simulink model "VSC_GFo_Variable_Frequency_LCL_r2015a"  (R2015a)
settings: Solver=ode1  SolverMode=SingleTasking  StartTime=0.0  StopTime=8  FixedStep=Time_Step  MaxStep=1e-5  RelTol=1e-3
PreLoadFcn:
  | VSC_GFo_Init;
InitFcn:
  | VSC_GFo_Init;
values from neighbouring files (symbols this model uses):
  DX_DR = 5    [VSC_GFo_Init.m]
  fb = fn    (= 50)    [VSC_GFo_Init.m]    (also in VSC_GFo_Init_v1.m; VSC_GFo_Init_wi_LCL.m)
  fn = 50    [VSC_GFo_Init.m]    (also in VSC_GFo_Init_v1.m; VSC_GFo_Init_wi_LCL.m)
  GRD00_Lg = GRD00_Xg/wb    (= 0.0254647908947)    [VSC_GFo_Init.m]    (also in VSC_GFo_Init_v1.m; VSC_GFo_Init_wi_LCL.m)
  GRD00_Rg = GRD00_Rg_pu*GRD00_Zb    (= 0.8)    [VSC_GFo_Init.m]    (also in VSC_GFo_Init_v1.m; VSC_GFo_Init_wi_LCL.m)
  I_thresh_pu = 1    [VSC_GFo_Init.m]
  Kp_Rvi_pu = 0.676    [VSC_GFo_Init.m]
  Time_Step = 40e-6    (= 4e-05)    [VSC_GFo_Init.m]    (also in VSC_GFo_Init_v1.m; VSC_GFo_Init_wi_LCL.m)
  VSC01_Delta_P_Time_Step = 0.2    [VSC_GFo_Init.m]    (also in VSC_GFo_Init_v1.m; VSC_GFo_Init_wi_LCL.m)
  VSC01_Delta_P_Value = 0    [VSC_GFo_Init.m]    (also in VSC_GFo_Init_v1.m = 0.2; VSC_GFo_Init_wi_LCL.m = 0.2)
  VSC01_Udc_n = 640 * 1e3    (= 640000)    [VSC_GFo_Init.m]    (also in VSC_GFo_Init_v1.m; VSC_GFo_Init_wi_LCL.m)
  VSC01_Udcb = VSC01_Udc_n    (= 640000)    [VSC_GFo_Init.m]    (also in VSC_GFo_Init_v1.m; VSC_GFo_Init_wi_LCL.m)
undefined symbols (not defined in the file or in its folder): C_line, powergui, VSC01_id0
undefined symbols (not defined in the file): GRD00_H, GRD00_R, GRD00_TD, GRD00_TN, GRD00_Ub, VSC01_Cf, VSC01_Cf_pu, VSC01_Lf, VSC01_Lf_pu, VSC01_Lt_pu, VSC01_mp1, VSC01_mp2, VSC01_mp3, VSC01_Pn, VSC01_R, VSC01_Rf, VSC01_Rf_pu, VSC01_Rt_pu, VSC01_Rv, VSC01_Sn, VSC01_T1, VSC01_T2, VSC01_Tr_PLL, VSC01_Un1, VSC01_Un2, VSC01_W_LF, VSC01_wc1, VSC01_wc2, VSC01_wc3
libraries: powerlib x28, simulink x1, powerlib_meascontrol x1
(part 2 of 2)

== system VSC_GFo_Variable_Frequency_LCL_r2015a/VSC00/Control loops/Inner Cascaded control loops ==
  eg_dq0* : Inport
  eg_dq : Inport  Port=2
  ig_dq : Inport  Port=3
  is_dq : Inport  Port=4
  Amplitude : Subsystem
  Compare To Constant : simulink/Logic and Bit Operations/Compare To Constant  relop=<=  const=I_max  OutDataTypeStr=boolean
  Current PI control : Subsystem
      mask Display:
      | plot(0,0,100,100, [10,10,90,90,10,40,40,10,90,60,60,90],[90,10,10,90,90,60,40,10,10,40,60,90])
      | disp('PI')
  Memory : Memory
  Voltage PI control : Subsystem
      mask Display:
      | plot(0,0,100,100, [10,10,90,90,10,40,40,10,90,60,60,90],[90,10,10,90,90,60,40,10,10,40,60,90])
      | disp('PI')
  w_pu : Constant
  vm_dq : Outport
  wires:
  Amplitude/2(cond) -> Compare To Constant/1
  eg_dq0*/1 -> Voltage PI control/2(Eg_dq0*)
  Voltage PI control/1(Is_dq0*) -> Amplitude/1(is_unsat)
  Amplitude/1(is_sat) -> Current PI control/3(Is_dq0*)
  w_pu/1 -> Current PI control/4(w), Voltage PI control/4(w)
  Current PI control/1(Vm_dq0*) -> vm_dq/1
  is_dq/1 -> Current PI control/1(Is_dq0)
  eg_dq/1 -> Current PI control/2(Eg_dq0), Voltage PI control/1(Eg_dq0)
  ig_dq/1 -> Voltage PI control/3(Ig_dq0)
  Compare To Constant/1 -> Memory/1
  Memory/1 -> Voltage PI control/5(block integ)

== system VSC_GFo_Variable_Frequency_LCL_r2015a/VSC00/Control loops/PLL ==
  vg_abc_pu : Inport
  Demux : Demux  Outputs=2
  PI PLL controller : Subsystem
  Terminator : Terminator
  abc --> dq (normalized) : Subsystem
  delta_PLL : Outport
  w_PLL : Outport  Port=2
  wires:
  Demux/2 -> PI PLL controller/1(Vq)
  PI PLL controller/1(w_PLL) -> w_PLL/1
  Demux/1 -> Terminator/1
  PI PLL controller/2(delta_theta) -> abc --> dq (normalized)/2(Theta), delta_PLL/1
  vg_abc_pu/1 -> abc --> dq (normalized)/1(abc)
  abc --> dq (normalized)/1(dq) -> Demux/1

== system VSC_GFo_Variable_Frequency_LCL_r2015a/VSC00/Control loops/Power Control Loops ==
  P_mes : Inport
  P_set : Inport  Port=2
  delta_PLL : Inport  Port=3
  w_PLL : Inport  Port=4
  Merge : Merge  Inputs=3
  Merge1 : Merge  Inputs=3
  Power control loops : Subsystem
  Strategy 1 : Subsystem
  Strategy 2 : Subsystem
  Switch Case : SwitchCase  CaseConditions={1,2,3}  ShowDefaultCase=off
  w_set2 : Constant  Value=gainpopup
  w_set_pu : Constant
  f : Outport
  Theta : Outport  Port=2
  wires:
  w_set2/1 -> Switch Case/1
  P_mes/1 -> Power control loops/1(P_mes), Strategy 2/1(P_mes), Strategy 1/1(P_mes)
  P_set/1 -> Strategy 2/2(P_set), Power control loops/2(P_set), Strategy 1/2(P_set)
  delta_PLL/1 -> Strategy 1/3(delta_PLL)
  w_PLL/1 -> Strategy 2/3(w_PLL), Strategy 1/4(w_PLL)
  Switch Case/1 -> Strategy 1/Action
  Switch Case/2 -> Strategy 2/Action
  w_set_pu/1 -> Power control loops/3(w_set_pu)
  Switch Case/3 -> Power control loops/Action
  Strategy 1/1(frequency) -> Merge/1
  Strategy 2/1(frequency) -> Merge/2
  Power control loops/1(frequency) -> Merge/3
  Strategy 1/2(theta) -> Merge1/1
  Strategy 2/2(theta) -> Merge1/2
  Power control loops/2(theta) -> Merge1/3
  Merge/1 -> f/1
  Merge1/1 -> Theta/1

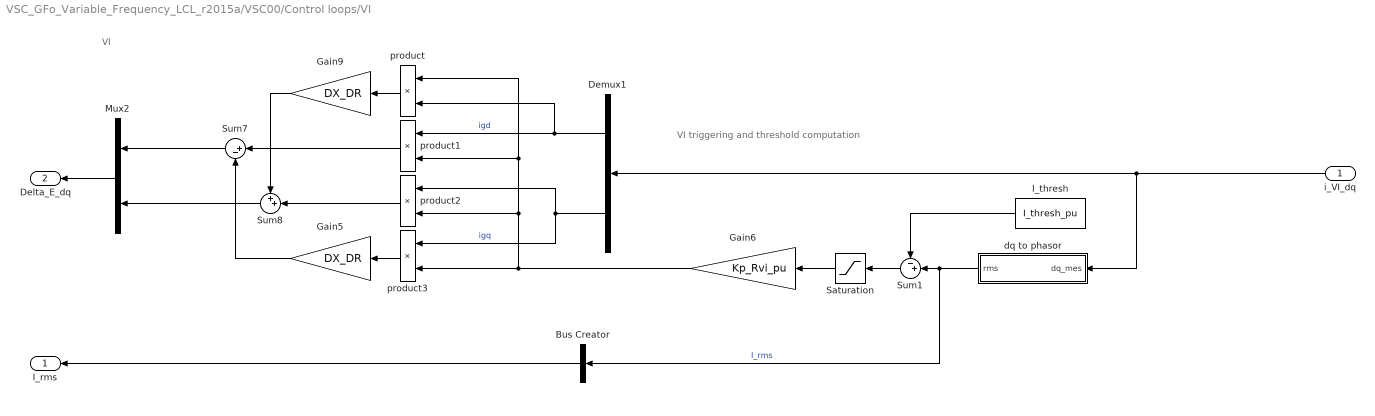
== system VSC_GFo_Variable_Frequency_LCL_r2015a/VSC00/Control loops/VI ==
  note: VI
  note: VI triggering and threshold computation
  i_VI_dq : Inport
  Bus Creator : BusCreator  Inputs=1
  Demux1 : Demux  Outputs=2
  Gain5 : Gain  Gain=DX_DR
  Gain6 : Gain  Gain=Kp_Rvi_pu
  Gain9 : Gain  Gain=DX_DR
  I_thresh : Constant  Value=I_thresh_pu
  Mux2 : Mux  Inputs=2
  Saturation : Saturate  UpperLimit=inf  LowerLimit=0
  Sum1 : Sum  Inputs=-+|
  Sum7 : Sum  Inputs=|+-
  Sum8 : Sum  Inputs=++|
  dq to phasor : Subsystem
  product{,1..3} (4 alike) : Product  SaturateOnIntegerOverflow=on  RndMeth=Zero  InputSameDT=on  OutDataTypeStr=Inherit: Same as first input
  I_rms : Outport
  Delta_E_dq : Outport  Port=2
  wires:
  i_VI_dq/1 -> Demux1/1, dq to phasor/1(dq_mes)
  Sum8/1 -> Mux2/2
  Sum7/1 -> Mux2/1
  product2/1 -> Sum8/2
  Gain9/1 -> Sum8/1
  Gain5/1 -> Sum7/2
  product1/1 -> Sum7/1
  Demux1/2 -> product3/1, product2/1  "igq"
  Demux1/1 -> product/2, product1/1  "igd"
  product/1 -> Gain9/1
  product3/1 -> Gain5/1
  Gain6/1 -> product2/2, product1/2, product/1, product3/2
  Mux2/1 -> Delta_E_dq/1
  I_thresh/1 -> Sum1/1
  Saturation/1 -> Gain6/1
  dq to phasor/1(rms) -> Bus Creator/1, Sum1/2  "I_rms"
  Sum1/1 -> Saturation/1
  Bus Creator/1 -> I_rms/1

== system VSC_GFo_Variable_Frequency_LCL_r2015a/VSC00/Control loops/abc --> dq (normalized) ==
  abc : Inport
  Theta : Inport  Port=2
  Demux3 : Demux  Outputs=3
  Mux2 : Mux  Inputs=2
  Normalization gain 1 pu rms in abc = 1 pu in dq : Gain  Gain=1/(sqrt(3))
  abc_2_alpha_beta : Subsystem
  alpha_beta_2_dq : Subsystem
  dq : Outport
  wires:
  Mux2/1 -> Normalization gain 1 pu rms in abc = 1 pu in dq/1
  abc_2_alpha_beta/1(alpha) -> alpha_beta_2_dq/2(a)
  Demux3/1 -> abc_2_alpha_beta/1(a)
  Demux3/2 -> abc_2_alpha_beta/2(b)
  alpha_beta_2_dq/1(d) -> Mux2/1
  abc_2_alpha_beta/2(beta) -> alpha_beta_2_dq/3(b)
  alpha_beta_2_dq/2(q) -> Mux2/2
  abc/1 -> Demux3/1
  Demux3/3 -> abc_2_alpha_beta/3(c)
  Theta/1 -> alpha_beta_2_dq/1(Theta)
  Normalization gain 1 pu rms in abc = 1 pu in dq/1 -> dq/1

== system VSC_GFo_Variable_Frequency_LCL_r2015a/VSC00/Control loops/abc --> dq (normalized)1 ==
  abc : Inport
  Theta : Inport  Port=2
  Demux3 : Demux  Outputs=3
  Mux2 : Mux  Inputs=2
  Normalization gain 1 pu rms in abc = 1 pu in dq : Gain  Gain=1/(sqrt(3))
  abc_2_alpha_beta : Subsystem
  alpha_beta_2_dq : Subsystem
  dq : Outport
  wires:
  Mux2/1 -> Normalization gain 1 pu rms in abc = 1 pu in dq/1
  abc_2_alpha_beta/1(alpha) -> alpha_beta_2_dq/2(a)
  Demux3/1 -> abc_2_alpha_beta/1(a)
  Demux3/2 -> abc_2_alpha_beta/2(b)
  alpha_beta_2_dq/1(d) -> Mux2/1
  abc_2_alpha_beta/2(beta) -> alpha_beta_2_dq/3(b)
  alpha_beta_2_dq/2(q) -> Mux2/2
  abc/1 -> Demux3/1
  Demux3/3 -> abc_2_alpha_beta/3(c)
  Theta/1 -> alpha_beta_2_dq/1(Theta)
  Normalization gain 1 pu rms in abc = 1 pu in dq/1 -> dq/1

== system VSC_GFo_Variable_Frequency_LCL_r2015a/VSC00/Control loops/abc --> dq (normalized)2 ==
  abc : Inport
  Theta : Inport  Port=2
  Demux3 : Demux  Outputs=3
  Mux2 : Mux  Inputs=2
  Normalization gain 1 pu rms in abc = 1 pu in dq : Gain  Gain=1/(sqrt(3))
  abc_2_alpha_beta : Subsystem
  alpha_beta_2_dq : Subsystem
  dq : Outport
  wires:
  Normalization gain 1 pu rms in abc = 1 pu in dq/1 -> dq/1
  Theta/1 -> alpha_beta_2_dq/1(Theta)
  Demux3/3 -> abc_2_alpha_beta/3(c)
  abc/1 -> Demux3/1
  alpha_beta_2_dq/2(q) -> Mux2/2
  abc_2_alpha_beta/2(beta) -> alpha_beta_2_dq/3(b)
  alpha_beta_2_dq/1(d) -> Mux2/1
  Demux3/2 -> abc_2_alpha_beta/2(b)
  Demux3/1 -> abc_2_alpha_beta/1(a)
  abc_2_alpha_beta/1(alpha) -> alpha_beta_2_dq/2(a)
  Mux2/1 -> Normalization gain 1 pu rms in abc = 1 pu in dq/1

== system VSC_GFo_Variable_Frequency_LCL_r2015a/VSC00/Control loops/dq  -->  abc (normalized) 1 ==
  dq : Inport
  Theta : Inport  Port=2
  Demux2 : Demux  Outputs=2
  Normalization gain 1 pu in dq = 1 pu rms in abc : Gain  Gain=sqrt(3)
  alpha_beta_2_abc : Subsystem
  dq_2_alpha_beta : Subsystem
  abc : Outport
  wires:
  Normalization gain 1 pu in dq = 1 pu rms in abc/1 -> Demux2/1
  alpha_beta_2_abc/1(abc) -> abc/1
  dq/1 -> Normalization gain 1 pu in dq = 1 pu rms in abc/1
  Theta/1 -> dq_2_alpha_beta/1(Theta)
  Demux2/2 -> dq_2_alpha_beta/3(q)
  Demux2/1 -> dq_2_alpha_beta/2(d)
  dq_2_alpha_beta/2(b) -> alpha_beta_2_abc/2(b)
  dq_2_alpha_beta/1(a) -> alpha_beta_2_abc/1(a)

== system VSC_GFo_Variable_Frequency_LCL_r2015a/powergui/EquivalentModel1/Gates ==
  Mux : Mux  Inputs=[1 1 1 1 1 1 1 1 1]
  gates : Outport
  wires:
  Mux/1 -> gates/1
  [T65_5966_6291969261697] -> Mux/1
  [T65_5964_6285887824649] -> Mux/2
  [T65_5965_6288835661788] -> Mux/3
  [T83_7448_10254691950676] -> Mux/4
  [T83_7449_10259102263635] -> Mux/5
  [T83_7450_10263758870811] -> Mux/6
  [T83_7449_10253676721795] -> Mux/7
  [T83_7450_10258084417385] -> Mux/8
  [T83_7451_10262738407191] -> Mux/9

== system VSC_GFo_Variable_Frequency_LCL_r2015a/powergui/EquivalentModel1/Sources ==
  Mux : Mux  Inputs=[2 1 1 1 1 1 3]
  Mux_u : Mux  Inputs=[9 10]
  SwitchCurrents : Constant  Value=zeros(9,1)
  u : Outport
  wires:
  Mux_u/1 -> u/1
  SwitchCurrents/1 -> Mux_u/1
  Mux/1 -> Mux_u/2
  [T67_6098_6569279523849] -> Mux/1
  [T72_6481_6701393223842] -> Mux/2
  [T59_5267_5517530445202] -> Mux/3
  [T97_9186_15014888992025] -> Mux/4
  [T97_9187_15014606156733] -> Mux/5
  [T97_9189_15014920846355] -> Mux/6
  [T71_6480_8065859831851] -> Mux/7

== system VSC_GFo_Variable_Frequency_LCL_r2015a/powergui/EquivalentModel1/Status ==
  status : Inport
  Demux : Demux  Outputs=[1 1 1 1 1 1 1 1 1]
  tag scope: T67_6199_7164623033795=global, T67_6200_7167043935260=global, T67_6201_7169645054337=global, T85_7683_11415309057765=global, T85_7684_11413922287263=global, T85_7684_11419160262613=global, T85_7685_11417770997179=global, T85_7685_11423251966521=global, T85_7686_11421860206154=global
  wires:
  status/1 -> Demux/1
  Demux/1 -> [T67_6201_7169645054337]
  Demux/2 -> [T67_6199_7164623033795]
  Demux/3 -> [T67_6200_7167043935260]
  Demux/4 -> [T85_7683_11415309057765]
  Demux/5 -> [T85_7684_11419160262613]
  Demux/6 -> [T85_7685_11423251966521]
  Demux/7 -> [T85_7684_11413922287263]
  Demux/8 -> [T85_7685_11417770997179]
  Demux/9 -> [T85_7686_11421860206154]

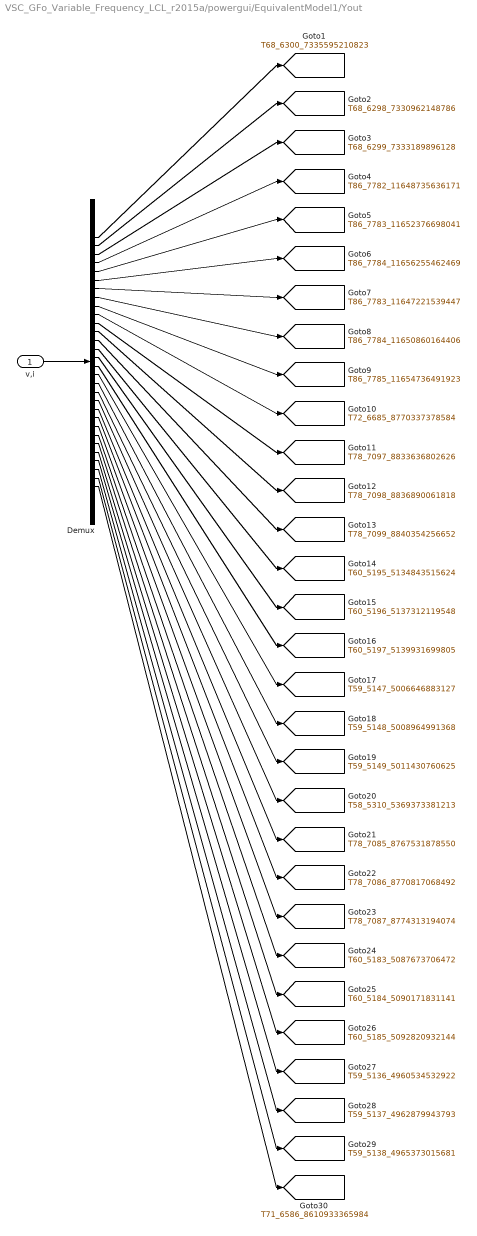
== system VSC_GFo_Variable_Frequency_LCL_r2015a/powergui/EquivalentModel1/Yout ==
  v,i : Inport
  Demux : Demux  Outputs=[1 1 1 1 1 1 1 1 1 1 1 1 1 1 1 1 1 1 1 1 1 1 1 1 1 1 1 1 1 2]
  tag scope: T58_5310_5369373381213=global, T59_5136_4960534532922=global, T59_5137_4962879943793=global, T59_5138_4965373015681=global, T59_5147_5006646883127=global, T59_5148_5008964991368=global, T59_5149_5011430760625=global, T60_5183_5087673706472=global, T60_5184_5090171831141=global, T60_5185_5092820932144=global, T60_5195_5134843515624=global, T60_5196_5137312119548=global, T60_5197_5139931699805=global, T68_6298_7330962148786=global, T68_6299_7333189896128=global, T68_6300_7335595210823=global, T71_6586_8610933365984=global, T72_6685_8770337378584=global, T78_7085_8767531878550=global, T78_7086_8770817068492=global, T78_7087_8774313194074=global, T78_7097_8833636802626=global, T78_7098_8836890061818=global, T78_7099_8840354256652=global, T86_7782_11648735636171=global, T86_7783_11647221539447=global, T86_7783_11652376698041=global, T86_7784_11650860164406=global, T86_7784_11656255462469=global, T86_7785_11654736491923=global
  wires:
  v,i/1 -> Demux/1
  Demux/1 -> [T68_6300_7335595210823]
  Demux/2 -> [T68_6298_7330962148786]
  Demux/3 -> [T68_6299_7333189896128]
  Demux/4 -> [T86_7782_11648735636171]
  Demux/5 -> [T86_7783_11652376698041]
  Demux/6 -> [T86_7784_11656255462469]
  Demux/7 -> [T86_7783_11647221539447]
  Demux/8 -> [T86_7784_11650860164406]
  Demux/9 -> [T86_7785_11654736491923]
  Demux/10 -> [T72_6685_8770337378584]
  Demux/11 -> [T78_7097_8833636802626]
  Demux/12 -> [T78_7098_8836890061818]
  Demux/13 -> [T78_7099_8840354256652]
  Demux/14 -> [T60_5195_5134843515624]
  Demux/15 -> [T60_5196_5137312119548]
  Demux/16 -> [T60_5197_5139931699805]
  Demux/17 -> [T59_5147_5006646883127]
  Demux/18 -> [T59_5148_5008964991368]
  Demux/19 -> [T59_5149_5011430760625]
  Demux/20 -> [T58_5310_5369373381213]
  Demux/21 -> [T78_7085_8767531878550]
  Demux/22 -> [T78_7086_8770817068492]
  Demux/23 -> [T78_7087_8774313194074]
  Demux/24 -> [T60_5183_5087673706472]
  Demux/25 -> [T60_5184_5090171831141]
  Demux/26 -> [T60_5185_5092820932144]
  Demux/27 -> [T59_5136_4960534532922]
  Demux/28 -> [T59_5137_4962879943793]
  Demux/29 -> [T59_5138_4965373015681]
  Demux/30 -> [T71_6586_8610933365984]

== system VSC_GFo_Variable_Frequency_LCL_r2015a/Inertial Voltage Source/Simplified SG/Power control1/Subsystem ==
  In1 : Inport
  Integrator3 : Integrator  InitialCondition=P0_VS*(1-TN/TD)
  Sum1 : Sum
  Sum2 : Sum  Inputs=+-
  mp1 : Gain  Gain=TN/TD
  mp2 : Gain  Gain=1-TN/TD
  mp3 : Gain  Gain=1/TD
  Out1 : Outport
  wires:
  Sum2/1 -> mp3/1
  mp3/1 -> Integrator3/1
  Integrator3/1 -> Sum1/2, Sum2/2
  In1/1 -> mp1/1, mp2/1
  mp2/1 -> Sum2/1
  mp1/1 -> Sum1/1
  Sum1/1 -> Out1/1

== system VSC_GFo_Variable_Frequency_LCL_r2015a/Inertial Voltage Source/Simplified SG/Power control1/dq  -->  abc  ==
  e_dq : Inport
  Theta : Inport  Port=2
  Demux2 : Demux  Outputs=2
  Scope1 : Scope
      settings: TimeRange=auto  MaxDataPoints=5000  SaveToWorkspace=off  SaveName=ScopeData11  YMin=-0.125  YMax=1.125  SampleTime=-1
  abc_alpha_beta : Subsystem
  abc_dq2 : Subsystem
  e_a_ref : Outport
  e_b_ref : Outport  Port=2
  e_c_ref : Outport  Port=3
  wires:
  abc_dq2/1(a) -> abc_alpha_beta/1(a)
  abc_dq2/2(b) -> abc_alpha_beta/2(b)
  Demux2/1 -> abc_dq2/2(d)
  Demux2/2 -> abc_dq2/3(q)
  Theta/1 -> abc_dq2/1(Theta)
  abc_alpha_beta/2(b1) -> e_b_ref/1
  e_dq/1 -> Demux2/1, Scope1/1
  abc_alpha_beta/3(c) -> e_c_ref/1
  abc_alpha_beta/1(a1) -> e_a_ref/1

== system VSC_GFo_Variable_Frequency_LCL_r2015a/VSC00/Control loops/Damping/Filter w_LF ==
  e : Inport
  1/T_LP : Gain  Gain=W_TVR  SaturateOnIntegerOverflow=on  OutDataTypeStr=Inherit: Same as input  ParamDataTypeStr=Inherit: Same as input
  Integrator : Integrator  InitialConditionSource=external  InitialCondition=[VSC01_id0*0.04]
  Sum1 : Sum  Inputs=|+-  SaturateOnIntegerOverflow=on  InputSameDT=on  OutDataTypeStr=Inherit: Same as first input
  s : Outport
  wires:
  Sum1/1 -> 1/T_LP/1
  1/T_LP/1 -> Integrator/1
  Integrator/1 -> Sum1/2, s/1
  e/1 -> Integrator/2, Sum1/1

== system VSC_GFo_Variable_Frequency_LCL_r2015a/VSC00/Control loops/Inner Cascaded control loops/Amplitude ==
  is_unsat : Inport
  Saturation2 : Saturate  UpperLimit=I_max  LowerLimit=0
  Source Element3 : Subsystem  AncestorBlock=simulink/REM/SE
  Subsystem : Subsystem
  dq to phasor : Subsystem
  is_sat : Outport
  cond : Outport  Port=2
  wires:
  dq to phasor/1(rms) -> cond/1, Saturation2/1
  Source Element3/1(ig_sat) -> is_sat/1
  Saturation2/1 -> Source Element3/1(Is_sat)
  Subsystem/1(phi) -> Source Element3/2(phi)
  is_unsat/1 -> dq to phasor/1(dq_mes), Subsystem/1(is_unsat)

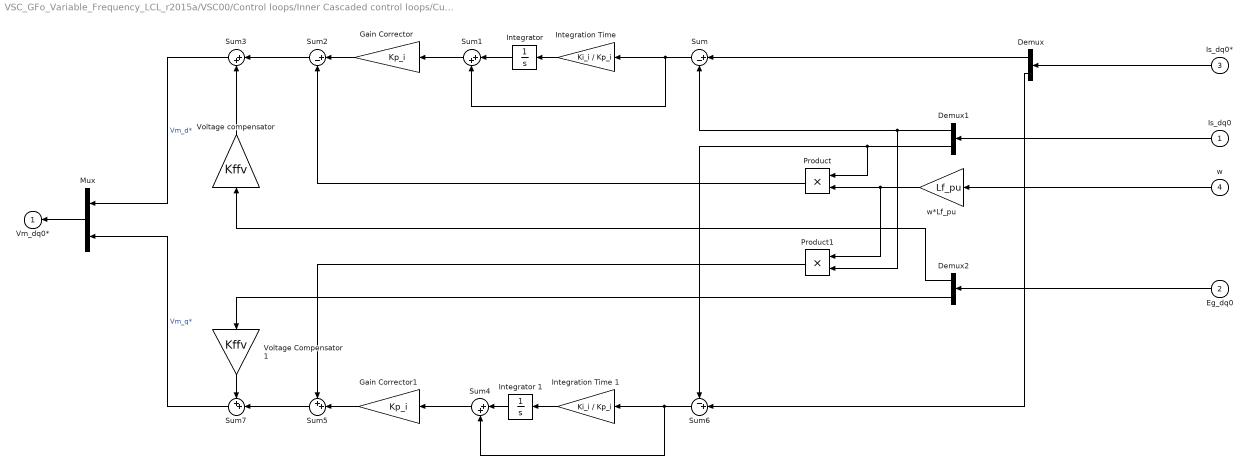
== system VSC_GFo_Variable_Frequency_LCL_r2015a/VSC00/Control loops/Inner Cascaded control loops/Current PI control ==
  Is_dq0 : Inport
  Eg_dq0 : Inport  Port=2
  Is_dq0* : Inport  Port=3
  w : Inport  Port=4
  Demux : Demux  Outputs=2
  Demux1 : Demux  Outputs=2
  Demux2 : Demux  Outputs=2
  Gain Corrector : Gain  Gain=Kp_i
  Gain Corrector1 : Gain  Gain=Kp_i
  Integration Time : Gain  Gain=Ki_i / Kp_i
  Integration Time 1 : Gain  Gain=Ki_i / Kp_i
  Integrator : Integrator
  Integrator 1 : Integrator
  Mux : Mux  Inputs=[1 1]
  Product : Product  RndMeth=Zero
  Product1 : Product  RndMeth=Zero
  Sum : Sum  Inputs=|+-
  Sum1 : Sum  Inputs=|++
  Sum2 : Sum  Inputs=|+-
  Sum3 : Sum  Inputs=|++
  Sum4 : Sum  Inputs=|++
  Sum5 : Sum  Inputs=++|
  Sum6 : Sum  Inputs=-+|
  Sum7 : Sum  Inputs=++|
  Voltage Compensator 1 : Gain  Gain=Kffv
  Voltage compensator : Gain  Gain=Kffv
  w*Lf_pu : Gain  Gain=Lf_pu
  Vm_dq0* : Outport  InitialOutput=0
  wires:
  Voltage Compensator 1/1 -> Sum7/1
  Voltage compensator/1 -> Sum3/2
  w/1 -> w*Lf_pu/1
  Integrator 1/1 -> Sum4/1
  Integrator/1 -> Sum1/1
  Integration Time/1 -> Integrator/1
  Sum/1 -> Integration Time/1, Sum1/2
  Sum4/1 -> Gain Corrector1/1
  Integration Time 1/1 -> Integrator 1/1
  Sum6/1 -> Integration Time 1/1, Sum4/2
  Sum7/1 -> Mux/2  "Vm_q*"
  Sum3/1 -> Mux/1  "Vm_d*"
  Sum5/1 -> Sum7/2
  Product1/1 -> Sum5/1
  Gain Corrector1/1 -> Sum5/2
  Demux/2 -> Sum6/2
  Mux/1 -> Vm_dq0*/1
  Sum2/1 -> Sum3/1
  Product/1 -> Sum2/2
  Demux1/2 -> Sum6/1, Product/1
  w*Lf_pu/1 -> Product/2, Product1/1
  Gain Corrector/1 -> Sum2/1
  Demux1/1 -> Sum/2, Product1/2
  Demux/1 -> Sum/1
  Sum1/1 -> Gain Corrector/1
  Is_dq0*/1 -> Demux/1
  Is_dq0/1 -> Demux1/1
  Demux2/1 -> Voltage compensator/1
  Demux2/2 -> Voltage Compensator 1/1
  Eg_dq0/1 -> Demux2/1

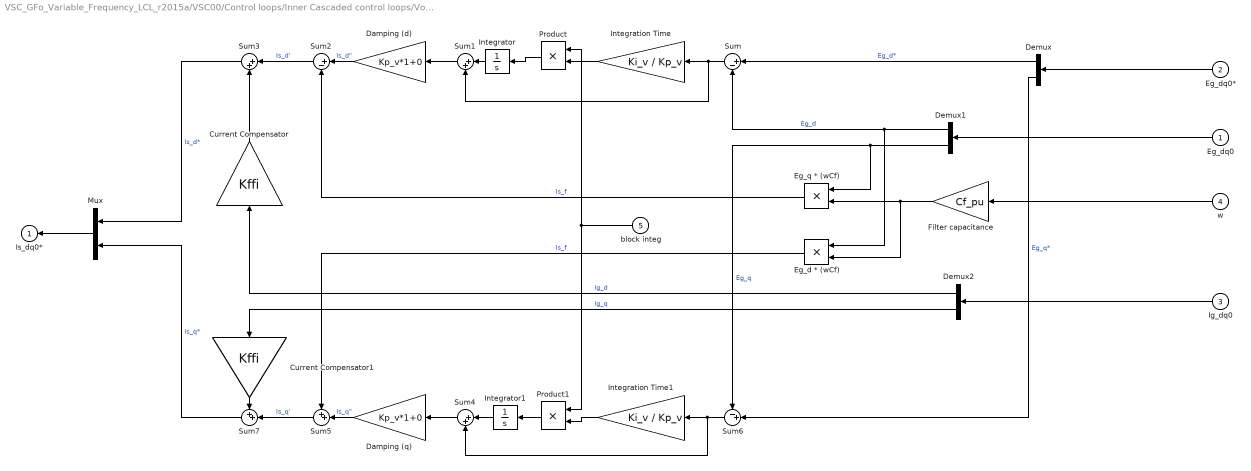
== system VSC_GFo_Variable_Frequency_LCL_r2015a/VSC00/Control loops/Inner Cascaded control loops/Voltage PI control ==
  Eg_dq0 : Inport
  Eg_dq0* : Inport  Port=2
  Ig_dq0 : Inport  Port=3
  w : Inport  Port=4
  block integ : Inport  Port=5
  Current Compensator : Gain  Gain=Kffi
  Current Compensator1 : Gain  Gain=Kffi
  Damping (d) : Gain  Gain=Kp_v*1+0
  Damping (q) : Gain  Gain=Kp_v*1+0
  Demux : Demux  Outputs=2
  Demux1 : Demux  Outputs=2
  Demux2 : Demux  Outputs=2
  Eg_d * (wCf) : Product  RndMeth=Zero
  "Eg_q * (wCf) " : Product  RndMeth=Zero
  Filter capacitance : Gain  Gain=Cf_pu
  Integration Time : Gain  Gain=Ki_v / Kp_v
  Integration Time1 : Gain  Gain=Ki_v / Kp_v
  Integrator : Integrator
  Integrator1 : Integrator
  Mux : Mux  Inputs=2
  Product : Product
  Product1 : Product
  Sum : Sum  Inputs=|+-
  Sum1 : Sum  Inputs=|++
  Sum2 : Sum  Inputs=|+-
  Sum3 : Sum  Inputs=|++
  Sum4 : Sum  Inputs=|++
  Sum5 : Sum  Inputs=++|
  Sum6 : Sum  Inputs=-+|
  Sum7 : Sum  Inputs=++|
  Is_dq0* : Outport  InitialOutput=0
  wires:
  Product1/1 -> Integrator1/1
  Product/1 -> Integrator/1
  block integ/1 -> Product/1, Product1/1
  Integration Time1/1 -> Product1/2
  Integration Time/1 -> Product/2
  Integrator1/1 -> Sum4/1
  Integrator/1 -> Sum1/1
  Current Compensator1/1 -> Sum7/1
  Current Compensator/1 -> Sum3/2
  w/1 -> Filter capacitance/1
  Sum7/1 -> Mux/2  "Is_q*"
  Sum3/1 -> Mux/1  "Is_d*"
  Sum5/1 -> Sum7/2  "Is_q'"
  Demux2/2 -> Current Compensator1/1  "Ig_q"
  Eg_d * (wCf)/1 -> Sum5/1  "Is_f"
  Damping (q)/1 -> Sum5/2  "Is_q\""
  Demux/2 -> Sum6/2  "Eg_q*"
  Sum4/1 -> Damping (q)/1
  Sum6/1 -> Integration Time1/1, Sum4/2
  Mux/1 -> Is_dq0*/1
  Demux2/1 -> Current Compensator/1  "Ig_d"
  Sum2/1 -> Sum3/1  "Is_d'"
  "Eg_q * (wCf) "/1 -> Sum2/2  "Is_f"
  Demux1/2 -> Sum6/1, "Eg_q * (wCf) "/1  "Eg_q"
  Filter capacitance/1 -> Eg_d * (wCf)/2, "Eg_q * (wCf) "/2
  Damping (d)/1 -> Sum2/1  "Is_d\""
  Demux1/1 -> Sum/2, Eg_d * (wCf)/1  "Eg_d"
  Demux/1 -> Sum/1  "Eg_d*"
  Sum1/1 -> Damping (d)/1
  Sum/1 -> Sum1/2, Integration Time/1
  Eg_dq0/1 -> Demux1/1
  Eg_dq0*/1 -> Demux/1
  Ig_dq0/1 -> Demux2/1

== system VSC_GFo_Variable_Frequency_LCL_r2015a/VSC00/Control loops/PLL/PI PLL controller ==
  Vq : Inport
  0 - Vd1 : Gain  Gain=Kp_PLL_pu  SaturateOnIntegerOverflow=on  OutDataTypeStr=Inherit: Same as input  ParamDataTypeStr=Inherit: Same as input
  0 - Vd2 : Gain  Gain=Ki_PLL_pu  SaturateOnIntegerOverflow=on  OutDataTypeStr=Inherit: Same as input  ParamDataTypeStr=Inherit: Same as input
  Integrator : Integrator
  Integrator1 : Integrator  InitialCondition=Theta0*pi/180
  Sum : Sum  SaturateOnIntegerOverflow=on
  Sum1 : Sum  SaturateOnIntegerOverflow=on
  w_PLL_pu : Gain  Gain=wb  SaturateOnIntegerOverflow=on  OutDataTypeStr=Inherit: Same as input  ParamDataTypeStr=Inherit: Same as input
  w_set : Constant
  w_PLL : Outport
  delta_theta : Outport  Port=2
  wires:
  0 - Vd2/1 -> Integrator/1
  w_set/1 -> Sum1/1
  w_PLL_pu/1 -> Integrator1/1
  Integrator/1 -> Sum/2
  Sum/1 -> Sum1/2
  0 - Vd1/1 -> Sum/1
  Vq/1 -> 0 - Vd2/1, 0 - Vd1/1
  Integrator1/1 -> delta_theta/1
  Sum1/1 -> w_PLL/1, w_PLL_pu/1

== system VSC_GFo_Variable_Frequency_LCL_r2015a/VSC00/Control loops/PLL/abc --> dq (normalized) ==
  abc : Inport
  Theta : Inport  Port=2
  Demux3 : Demux  Outputs=3
  Mux2 : Mux  Inputs=2
  Normalization gain 1 pu rms in abc = 1 pu in dq : Gain  Gain=1/(sqrt(3))
  abc_2_alpha_beta : Subsystem
  alpha_beta_2_dq : Subsystem
  dq : Outport
  wires:
  Mux2/1 -> Normalization gain 1 pu rms in abc = 1 pu in dq/1
  abc_2_alpha_beta/1(alpha) -> alpha_beta_2_dq/2(a)
  Demux3/1 -> abc_2_alpha_beta/1(a)
  Demux3/2 -> abc_2_alpha_beta/2(b)
  alpha_beta_2_dq/1(d) -> Mux2/1
  abc_2_alpha_beta/2(beta) -> alpha_beta_2_dq/3(b)
  alpha_beta_2_dq/2(q) -> Mux2/2
  abc/1 -> Demux3/1
  Demux3/3 -> abc_2_alpha_beta/3(c)
  Theta/1 -> alpha_beta_2_dq/1(Theta)
  Normalization gain 1 pu rms in abc = 1 pu in dq/1 -> dq/1

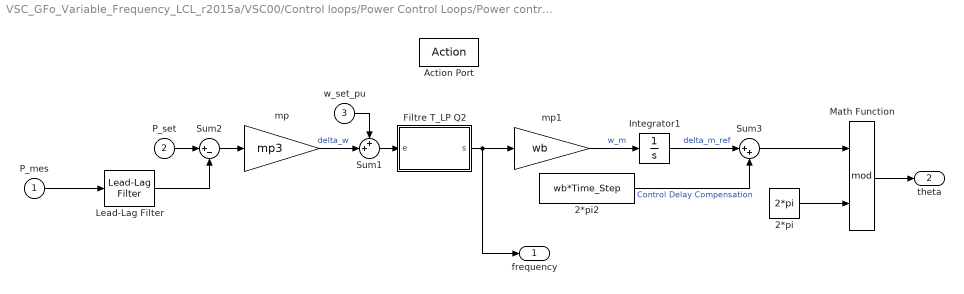
== system VSC_GFo_Variable_Frequency_LCL_r2015a/VSC00/Control loops/Power Control Loops/Power control loops ==
  P_mes : Inport
  P_set : Inport  Port=2
  w_set_pu : Inport  Port=3
  Action Port : ActionPort  ActionType=case
  2*pi : Constant  Value=2*pi
  2*pi2 : Constant  Value=wb*Time_Step
  Filtre T_LP Q2 : Subsystem
  Integrator1 : Integrator  InitialCondition=Theta_vsc0*pi/180
  Lead-Lag Filter : powerlib_meascontrol/Filters/Lead-Lag Filter  T1=T1  T2=T2  Vdc_Init=P0  Ts=0
  Math Function : Math  Operator=mod  SaturateOnIntegerOverflow=on
  Sum1 : Sum  Inputs=++|
  Sum2 : Sum  Inputs=|+-
  Sum3 : Sum  Inputs=|++
  mp : Gain  Gain=mp3
  mp1 : Gain  Gain=wb
  frequency : Outport
  theta : Outport  Port=2
  wires:
  Sum2/1 -> mp/1
  Integrator1/1 -> Sum3/1  "delta_m_ref"
  Math Function/1 -> theta/1
  2*pi/1 -> Math Function/2
  w_set_pu/1 -> Sum1/1
  P_set/1 -> Sum2/1
  mp/1 -> Sum1/2  "delta_w"
  Filtre T_LP Q2/1(s) -> frequency/1, mp1/1
  P_mes/1 -> Lead-Lag Filter/1
  Sum1/1 -> Filtre T_LP Q2/1(e)
  mp1/1 -> Integrator1/1  "w_m"
  Sum3/1 -> Math Function/1
  2*pi2/1 -> Sum3/2  "Control Delay Compensation"
  Lead-Lag Filter/1 -> Sum2/2

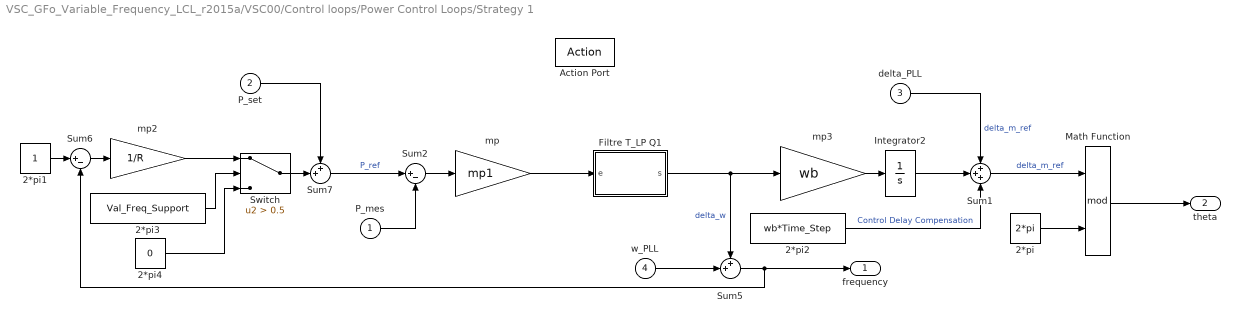
== system VSC_GFo_Variable_Frequency_LCL_r2015a/VSC00/Control loops/Power Control Loops/Strategy 1 ==
  P_mes : Inport
  P_set : Inport  Port=2
  delta_PLL : Inport  Port=3
  w_PLL : Inport  Port=4
  Action Port : ActionPort  ActionType=case
  2*pi : Constant  Value=2*pi
  2*pi1 : Constant
  2*pi2 : Constant  Value=wb*Time_Step
  2*pi3 : Constant  Value=Val_Freq_Support
  2*pi4 : Constant  Value=0
  Filtre T_LP Q1 : Subsystem
  Integrator2 : Integrator  InitialCondition=(Theta_vsc0-Theta0)*pi/180
  Math Function : Math  Operator=mod  SaturateOnIntegerOverflow=on
  Sum1 : Sum  Inputs=+++
  Sum2 : Sum  Inputs=|+-
  Sum5 : Sum  Inputs=++|
  Sum6 : Sum  Inputs=|+-
  Sum7 : Sum  Inputs=++|
  Switch : Switch  Criteria=u2 > Threshold  Threshold=0.5
  mp : Gain  Gain=mp1
  mp2 : Gain  Gain=1/R
  mp3 : Gain  Gain=wb
  frequency : Outport
  theta : Outport  Port=2
  wires:
  Sum2/1 -> mp/1
  Sum1/1 -> Math Function/1  "delta_m_ref"
  2*pi/1 -> Math Function/2
  2*pi1/1 -> Sum6/1
  Sum6/1 -> mp2/1
  P_set/1 -> Sum7/1
  Sum7/1 -> Sum2/1  "P_ref"
  P_mes/1 -> Sum2/2
  Switch/1 -> Sum7/2
  Math Function/1 -> theta/1
  Filtre T_LP Q1/1(s) -> mp3/1, Sum5/1  "delta_w"
  mp3/1 -> Integrator2/1
  mp/1 -> Filtre T_LP Q1/1(e)
  delta_PLL/1 -> Sum1/1  "delta_m_ref"
  w_PLL/1 -> Sum5/2
  Sum5/1 -> frequency/1, Sum6/2
  2*pi2/1 -> Sum1/3  "Control Delay Compensation"
  Integrator2/1 -> Sum1/2
  mp2/1 -> Switch/1
  2*pi3/1 -> Switch/2
  2*pi4/1 -> Switch/3

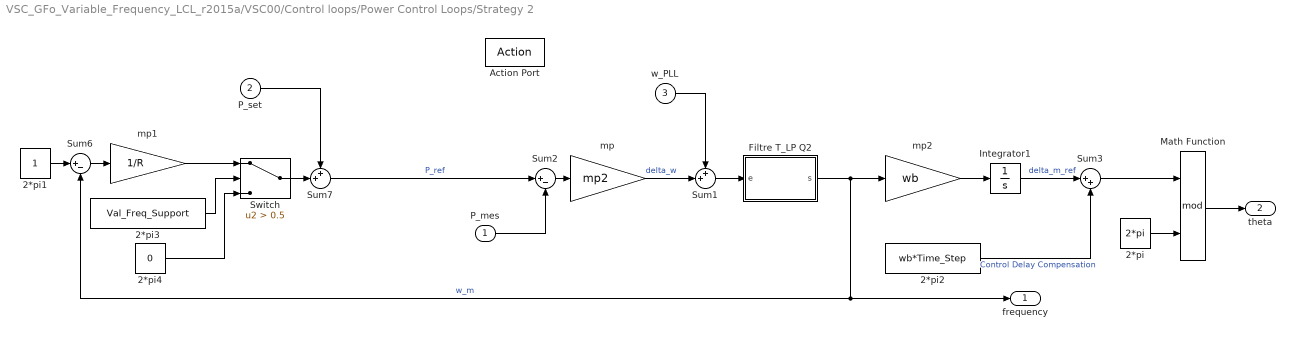
== system VSC_GFo_Variable_Frequency_LCL_r2015a/VSC00/Control loops/Power Control Loops/Strategy 2 ==
  P_mes : Inport
  P_set : Inport  Port=2
  w_PLL : Inport  Port=3
  Action Port : ActionPort  ActionType=case
  2*pi : Constant  Value=2*pi
  2*pi1 : Constant
  2*pi2 : Constant  Value=wb*Time_Step
  2*pi3 : Constant  Value=Val_Freq_Support
  2*pi4 : Constant  Value=0
  Filtre T_LP Q2 : Subsystem
  Integrator1 : Integrator  InitialCondition=Theta_vsc0*pi/180
  Math Function : Math  Operator=mod  SaturateOnIntegerOverflow=on
  Sum1 : Sum  Inputs=++|
  Sum2 : Sum  Inputs=|+-
  Sum3 : Sum  Inputs=|++
  Sum6 : Sum  Inputs=|+-
  Sum7 : Sum  Inputs=++|
  Switch : Switch  Criteria=u2 > Threshold  Threshold=0.5
  mp : Gain  Gain=mp2
  mp1 : Gain  Gain=1/R
  mp2 : Gain  Gain=wb
  frequency : Outport
  theta : Outport  Port=2
  wires:
  Sum1/1 -> Filtre T_LP Q2/1(e)
  2*pi/1 -> Math Function/2
  Math Function/1 -> theta/1
  Integrator1/1 -> Sum3/1  "delta_m_ref"
  Sum2/1 -> mp/1
  mp/1 -> Sum1/2  "delta_w"
  Filtre T_LP Q2/1(s) -> mp2/1, frequency/1, Sum6/2  "w_m"
  w_PLL/1 -> Sum1/1
  P_mes/1 -> Sum2/2
  mp2/1 -> Integrator1/1
  2*pi2/1 -> Sum3/2  "Control Delay Compensation"
  Sum3/1 -> Math Function/1
  Switch/1 -> Sum7/2
  P_set/1 -> Sum7/1
  Sum6/1 -> mp1/1
  2*pi1/1 -> Sum6/1
  mp1/1 -> Switch/1
  2*pi3/1 -> Switch/2
  2*pi4/1 -> Switch/3
  Sum7/1 -> Sum2/1  "P_ref"

== system VSC_GFo_Variable_Frequency_LCL_r2015a/VSC00/Control loops/VI/dq to phasor ==
  dq_mes : Inport
  Demux : Demux  Outputs=2
  Sqrt : Sqrt  SaturateOnIntegerOverflow=on
  Sum4 : Sum  Inputs=|++  SaturateOnIntegerOverflow=on  InputSameDT=on  OutDataTypeStr=Inherit: Same as first input
  Vrdird : Product  SaturateOnIntegerOverflow=on  RndMeth=Zero  InputSameDT=on  OutDataTypeStr=Inherit: Same as first input
  Vrqirq : Product  SaturateOnIntegerOverflow=on  RndMeth=Zero  InputSameDT=on  OutDataTypeStr=Inherit: Same as first input
  rms : Outport
  wires:
  Sqrt/1 -> rms/1
  dq_mes/1 -> Demux/1
  Demux/1 -> Vrdird/1, Vrdird/2
  Demux/2 -> Vrqirq/1, Vrqirq/2
  Vrdird/1 -> Sum4/1
  Vrqirq/1 -> Sum4/2
  Sum4/1 -> Sqrt/1

== system VSC_GFo_Variable_Frequency_LCL_r2015a/VSC00/Control loops/abc --> dq (normalized)/abc_2_alpha_beta ==
  a : Inport
  b : Inport  Port=2
  c : Inport  Port=3
  Fcn1 : Fcn  Expr=sqrt(2/3)*(u(1)+u(2)+u(3))
  Fcn3 : Fcn  Expr=sqrt(2/3)*(u(1)-u(2)/2-u(3)/2)
  Fcn5 : Fcn  Expr=(u(2)-u(3))/sqrt(2)
  Mux : Mux  Inputs=3
  Scope5 : Scope
      settings: TimeRange=auto  MaxDataPoints=5000  SaveToWorkspace=off  SaveName=ScopeData17  YMin=0  YMax=425  SampleTime=-1
  alpha : Outport
  beta : Outport  Port=2
  wires:
  c/1 -> Mux/3
  Fcn1/1 -> Scope5/1
  Mux/1 -> Fcn1/1, Fcn3/1, Fcn5/1
  a/1 -> Mux/1
  b/1 -> Mux/2
  Fcn3/1 -> alpha/1
  Fcn5/1 -> beta/1

== system VSC_GFo_Variable_Frequency_LCL_r2015a/VSC00/Control loops/abc --> dq (normalized)/alpha_beta_2_dq ==
  Theta : Inport
  a : Inport  Port=2
  b : Inport  Port=3
  Fcn1 : Fcn  Expr=u(2)*cos(u(1))+u(3)*sin(u(1))
  Fcn3 : Fcn  Expr=u(2)*sin(u(1))-u(3)*cos(u(1))
  Mux : Mux  Inputs=3
  d : Outport
  q : Outport  Port=2
  wires:
  Theta/1 -> Mux/1
  Mux/1 -> Fcn3/1, Fcn1/1
  a/1 -> Mux/2
  b/1 -> Mux/3
  Fcn3/1 -> d/1
  Fcn1/1 -> q/1

== system VSC_GFo_Variable_Frequency_LCL_r2015a/VSC00/Control loops/abc --> dq (normalized)1/abc_2_alpha_beta ==
  a : Inport
  b : Inport  Port=2
  c : Inport  Port=3
  Fcn1 : Fcn  Expr=sqrt(2/3)*(u(1)+u(2)+u(3))
  Fcn3 : Fcn  Expr=sqrt(2/3)*(u(1)-u(2)/2-u(3)/2)
  Fcn5 : Fcn  Expr=(u(2)-u(3))/sqrt(2)
  Mux : Mux  Inputs=3
  Scope5 : Scope
      settings: TimeRange=auto  MaxDataPoints=5000  SaveToWorkspace=off  SaveName=ScopeData17  YMin=0  YMax=425  SampleTime=-1
  alpha : Outport
  beta : Outport  Port=2
  wires:
  c/1 -> Mux/3
  Fcn1/1 -> Scope5/1
  Mux/1 -> Fcn1/1, Fcn3/1, Fcn5/1
  a/1 -> Mux/1
  b/1 -> Mux/2
  Fcn3/1 -> alpha/1
  Fcn5/1 -> beta/1

== system VSC_GFo_Variable_Frequency_LCL_r2015a/VSC00/Control loops/abc --> dq (normalized)1/alpha_beta_2_dq ==
  Theta : Inport
  a : Inport  Port=2
  b : Inport  Port=3
  Fcn1 : Fcn  Expr=u(2)*cos(u(1))+u(3)*sin(u(1))
  Fcn3 : Fcn  Expr=u(2)*sin(u(1))-u(3)*cos(u(1))
  Mux : Mux  Inputs=3
  d : Outport
  q : Outport  Port=2
  wires:
  Theta/1 -> Mux/1
  Mux/1 -> Fcn3/1, Fcn1/1
  a/1 -> Mux/2
  b/1 -> Mux/3
  Fcn3/1 -> d/1
  Fcn1/1 -> q/1

== system VSC_GFo_Variable_Frequency_LCL_r2015a/VSC00/Control loops/abc --> dq (normalized)2/abc_2_alpha_beta ==
  a : Inport
  b : Inport  Port=2
  c : Inport  Port=3
  Fcn1 : Fcn  Expr=sqrt(2/3)*(u(1)+u(2)+u(3))
  Fcn3 : Fcn  Expr=sqrt(2/3)*(u(1)-u(2)/2-u(3)/2)
  Fcn5 : Fcn  Expr=(u(2)-u(3))/sqrt(2)
  Mux : Mux  Inputs=3
  Scope5 : Scope
      settings: TimeRange=auto  MaxDataPoints=5000  SaveToWorkspace=off  SaveName=ScopeData17  YMin=0  YMax=425  SampleTime=-1
  alpha : Outport
  beta : Outport  Port=2
  wires:
  Fcn5/1 -> beta/1
  Fcn3/1 -> alpha/1
  b/1 -> Mux/2
  a/1 -> Mux/1
  Mux/1 -> Fcn5/1, Fcn3/1, Fcn1/1
  Fcn1/1 -> Scope5/1
  c/1 -> Mux/3

== system VSC_GFo_Variable_Frequency_LCL_r2015a/VSC00/Control loops/abc --> dq (normalized)2/alpha_beta_2_dq ==
  Theta : Inport
  a : Inport  Port=2
  b : Inport  Port=3
  Fcn1 : Fcn  Expr=u(2)*cos(u(1))+u(3)*sin(u(1))
  Fcn3 : Fcn  Expr=u(2)*sin(u(1))-u(3)*cos(u(1))
  Mux : Mux  Inputs=3
  d : Outport
  q : Outport  Port=2
  wires:
  Fcn1/1 -> q/1
  Fcn3/1 -> d/1
  b/1 -> Mux/3
  a/1 -> Mux/2
  Mux/1 -> Fcn1/1, Fcn3/1
  Theta/1 -> Mux/1

== system VSC_GFo_Variable_Frequency_LCL_r2015a/VSC00/Control loops/dq  -->  abc (normalized) 1/alpha_beta_2_abc ==
  a : Inport
  b : Inport  Port=2
  Fcn1 : Fcn  Expr=(-u(1)-sqrt(3)*u(2))/2
  Fcn3 : Fcn  Expr=u(1)
  Fcn5 : Fcn  Expr=(-u(1)+sqrt(3)*u(2))/2
  Gain1 : Gain  Gain=sqrt(2/3)
  Gain2 : Gain  Gain=sqrt(2/3)
  Gain3 : Gain  Gain=sqrt(2/3)
  Mux : Mux  Inputs=2
  Mux1 : Mux  Inputs=[1 1 1]
  abc : Outport
  wires:
  Mux1/1 -> abc/1
  Gain3/1 -> Mux1/1
  Gain2/1 -> Mux1/2
  Gain1/1 -> Mux1/3
  Fcn1/1 -> Gain1/1
  Fcn5/1 -> Gain2/1
  Fcn3/1 -> Gain3/1
  b/1 -> Mux/2
  a/1 -> Mux/1
  Mux/1 -> Fcn1/1, Fcn5/1, Fcn3/1

== system VSC_GFo_Variable_Frequency_LCL_r2015a/VSC00/Control loops/dq  -->  abc (normalized) 1/dq_2_alpha_beta ==
  Theta : Inport
  d : Inport  Port=2
  q : Inport  Port=3
  Fcn1 : Fcn  Expr=-u(2)*cos(u(1))+u(3)*sin(u(1))
  Fcn3 : Fcn  Expr=u(2)*sin(u(1))+u(3)*cos(u(1))
  Mux : Mux  Inputs=3
  a : Outport
  b : Outport  Port=2
  wires:
  Mux/1 -> Fcn1/1, Fcn3/1
  Theta/1 -> Mux/1
  d/1 -> Mux/2
  q/1 -> Mux/3
  Fcn3/1 -> a/1
  Fcn1/1 -> b/1

== system VSC_GFo_Variable_Frequency_LCL_r2015a/Inertial Voltage Source/Simplified SG/Power control1/dq  -->  abc /abc_alpha_beta ==
  a : Inport
  b : Inport  Port=2
  Fcn1 : Fcn  Expr=(-u(1)-sqrt(3)*u(2))/2
  Fcn3 : Fcn  Expr=u(1)
  Fcn5 : Fcn  Expr=(-u(1)+sqrt(3)*u(2))/2
  Gain1 : Gain  Gain=sqrt(2)
  Gain2 : Gain  Gain=sqrt(2)
  Gain3 : Gain  Gain=sqrt(2)
  Mux : Mux  Inputs=2
  a1 : Outport
  b1 : Outport  Port=2
  c : Outport  Port=3
  wires:
  Mux/1 -> Fcn5/1, Fcn1/1, Fcn3/1
  a/1 -> Mux/1
  b/1 -> Mux/2
  Fcn3/1 -> Gain3/1
  Fcn5/1 -> Gain2/1
  Fcn1/1 -> Gain1/1
  Gain1/1 -> c/1
  Gain2/1 -> b1/1
  Gain3/1 -> a1/1

== system VSC_GFo_Variable_Frequency_LCL_r2015a/Inertial Voltage Source/Simplified SG/Power control1/dq  -->  abc /abc_dq2 ==
  Theta : Inport
  d : Inport  Port=2
  q : Inport  Port=3
  Fcn1 : Fcn  Expr=-u(2)*cos(u(1))+u(3)*sin(u(1))
  Fcn3 : Fcn  Expr=u(2)*sin(u(1))+u(3)*cos(u(1))
  Mux : Mux  Inputs=3
  a : Outport
  b : Outport  Port=2
  wires:
  Fcn1/1 -> b/1
  Fcn3/1 -> a/1
  q/1 -> Mux/3
  d/1 -> Mux/2
  Theta/1 -> Mux/1
  Mux/1 -> Fcn3/1, Fcn1/1

== system VSC_GFo_Variable_Frequency_LCL_r2015a/VSC00/Control loops/Inner Cascaded control loops/Amplitude/Source Element3 ==
  Is_sat : Inport
  phi : Inport  Port=2
  Mux : Mux  Inputs=2
  Product : Product
  Product1 : Product
  Trigonometric Function : Trigonometry  Operator=cos
  Trigonometric Function1 : Trigonometry
  ig_sat : Outport  InitialOutput=0
  wires:
  Is_sat/1 -> Product1/1, Product/1
  phi/1 -> Trigonometric Function1/1, Trigonometric Function/1
  Product/1 -> Mux/1
  Product1/1 -> Mux/2
  Mux/1 -> ig_sat/1
  Trigonometric Function1/1 -> Product1/2
  Trigonometric Function/1 -> Product/2

== system VSC_GFo_Variable_Frequency_LCL_r2015a/VSC00/Control loops/Inner Cascaded control loops/Amplitude/Subsystem ==
  is_unsat : Inport
  Demux2 : Demux  Outputs=2
  Trigonometric Function : Trigonometry  Operator=atan2  NumberOfIterations=5  OutputSignalType=real
  phi : Outport
  wires:
  Demux2/2 -> Trigonometric Function/1
  Trigonometric Function/1 -> phi/1
  Demux2/1 -> Trigonometric Function/2
  is_unsat/1 -> Demux2/1

== system VSC_GFo_Variable_Frequency_LCL_r2015a/VSC00/Control loops/Inner Cascaded control loops/Amplitude/dq to phasor ==
  dq_mes : Inport
  Demux : Demux  Outputs=2
  Sqrt : Sqrt  SaturateOnIntegerOverflow=on
  Sum4 : Sum  Inputs=|++  SaturateOnIntegerOverflow=on  InputSameDT=on  OutDataTypeStr=Inherit: Same as first input
  Vrdird : Product  SaturateOnIntegerOverflow=on  RndMeth=Zero  InputSameDT=on  OutDataTypeStr=Inherit: Same as first input
  Vrqirq : Product  SaturateOnIntegerOverflow=on  RndMeth=Zero  InputSameDT=on  OutDataTypeStr=Inherit: Same as first input
  rms : Outport
  wires:
  Sqrt/1 -> rms/1
  dq_mes/1 -> Demux/1
  Demux/1 -> Vrdird/1, Vrdird/2
  Demux/2 -> Vrqirq/1, Vrqirq/2
  Vrdird/1 -> Sum4/1
  Vrqirq/1 -> Sum4/2
  Sum4/1 -> Sqrt/1

== system VSC_GFo_Variable_Frequency_LCL_r2015a/VSC00/Control loops/PLL/abc --> dq (normalized)/abc_2_alpha_beta ==
  a : Inport
  b : Inport  Port=2
  c : Inport  Port=3
  Fcn1 : Fcn  Expr=sqrt(2/3)*(u(1)+u(2)+u(3))
  Fcn3 : Fcn  Expr=sqrt(2/3)*(u(1)-u(2)/2-u(3)/2)
  Fcn5 : Fcn  Expr=(u(2)-u(3))/sqrt(2)
  Mux : Mux  Inputs=3
  Scope5 : Scope
      settings: TimeRange=auto  MaxDataPoints=5000  SaveToWorkspace=off  SaveName=ScopeData17  YMin=0  YMax=425  SampleTime=-1
  alpha : Outport
  beta : Outport  Port=2
  wires:
  c/1 -> Mux/3
  Fcn1/1 -> Scope5/1
  Mux/1 -> Fcn1/1, Fcn3/1, Fcn5/1
  a/1 -> Mux/1
  b/1 -> Mux/2
  Fcn3/1 -> alpha/1
  Fcn5/1 -> beta/1

== system VSC_GFo_Variable_Frequency_LCL_r2015a/VSC00/Control loops/PLL/abc --> dq (normalized)/alpha_beta_2_dq ==
  Theta : Inport
  a : Inport  Port=2
  b : Inport  Port=3
  Fcn1 : Fcn  Expr=u(2)*cos(u(1))+u(3)*sin(u(1))
  Fcn3 : Fcn  Expr=u(2)*sin(u(1))-u(3)*cos(u(1))
  Mux : Mux  Inputs=3
  d : Outport
  q : Outport  Port=2
  wires:
  Theta/1 -> Mux/1
  Mux/1 -> Fcn3/1, Fcn1/1
  a/1 -> Mux/2
  b/1 -> Mux/3
  Fcn3/1 -> d/1
  Fcn1/1 -> q/1

== system VSC_GFo_Variable_Frequency_LCL_r2015a/VSC00/Control loops/Power Control Loops/Power control loops/Filtre T_LP Q2 ==
  e : Inport
  1/T_LP : Gain  Gain=wc3  SaturateOnIntegerOverflow=on  OutDataTypeStr=Inherit: Same as input  ParamDataTypeStr=Inherit: Same as input
  Integrator : Integrator  InitialCondition=1
  Sum1 : Sum  Inputs=|+-  SaturateOnIntegerOverflow=on  InputSameDT=on  OutDataTypeStr=Inherit: Same as first input
  s : Outport
  wires:
  Sum1/1 -> 1/T_LP/1
  1/T_LP/1 -> Integrator/1
  Integrator/1 -> Sum1/2, s/1
  e/1 -> Sum1/1

== system VSC_GFo_Variable_Frequency_LCL_r2015a/VSC00/Control loops/Power Control Loops/Strategy 1/Filtre T_LP Q1 ==
  e : Inport
  1/T_LP : Gain  Gain=wc1  SaturateOnIntegerOverflow=on  OutDataTypeStr=Inherit: Same as input  ParamDataTypeStr=Inherit: Same as input
  Integrator : Integrator
  Sum1 : Sum  Inputs=|+-  SaturateOnIntegerOverflow=on  InputSameDT=on  OutDataTypeStr=Inherit: Same as first input
  s : Outport
  wires:
  Sum1/1 -> 1/T_LP/1
  1/T_LP/1 -> Integrator/1
  Integrator/1 -> Sum1/2, s/1
  e/1 -> Sum1/1

== system VSC_GFo_Variable_Frequency_LCL_r2015a/VSC00/Control loops/Power Control Loops/Strategy 2/Filtre T_LP Q2 ==
  e : Inport
  1/T_LP : Gain  Gain=wc2  SaturateOnIntegerOverflow=on  OutDataTypeStr=Inherit: Same as input  ParamDataTypeStr=Inherit: Same as input
  Integrator : Integrator  InitialCondition=1
  Sum1 : Sum  Inputs=|+-  SaturateOnIntegerOverflow=on  InputSameDT=on  OutDataTypeStr=Inherit: Same as first input
  s : Outport
  wires:
  Sum1/1 -> 1/T_LP/1
  1/T_LP/1 -> Integrator/1
  Integrator/1 -> Sum1/2, s/1
  e/1 -> Sum1/1
